simulink model "Subsystem"  (R2020b)
settings: Solver=VariableStepAuto  StartTime=0.0  StopTime=10.0  RelTol=1e-3
settings Model: Creator=HP  LastModifiedBy=HP
settings DataIOCC: SaveOutput=off  SaveTime=off

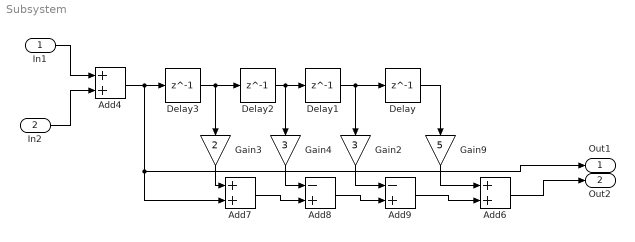
== system Subsystem ==
  In1 : Inport  OutDataTypeStr=double  PortDimensions=1  SampleTime=0
  In2 : Inport  Port=2  OutDataTypeStr=double  PortDimensions=1  SampleTime=0
  Add4 : Sum
  Add6 : Sum
  Add7 : Sum
  Add8 : Sum  Inputs=-+
  Add9 : Sum  Inputs=-+
  Delay{,1..3} (4 alike) : Delay  DelayLength=1
  Gain2 : Gain  Gain=3
  Gain3 : Gain  Gain=2
  Gain4 : Gain  Gain=3
  Gain9 : Gain  Gain=5
  Out1 : Outport  OutDataTypeStr=double  PortDimensions=1  SampleTime=0
  Out2 : Outport  Port=2  OutDataTypeStr=double  PortDimensions=1  SampleTime=0
  wires:
  Gain2/1 -> Add9/1
  Delay3/1 -> Gain3/1, Delay2/1
  Gain9/1 -> Add6/1
  In2/1 -> Add4/2
  In1/1 -> Add4/1
  Add8/1 -> Add9/2
  Gain4/1 -> Add8/1
  Delay/1 -> Gain9/1
  Delay2/1 -> Delay1/1, Gain4/1
  Add9/1 -> Add6/2
  Gain3/1 -> Add7/1
  Add7/1 -> Add8/2
  Add4/1 -> Add7/2, Out1/1, Delay3/1
  Delay1/1 -> Gain2/1, Delay/1
  Add6/1 -> Out2/1
